simulink model "untitled1"  (R2017b)
settings: Solver=ode4  StartTime=0.0  StopTime=6  FixedStep=Ts  RelTol=1e-3  EnableMultiTasking=on
values from neighbouring files (symbols this model uses):
  init = []    [tunning.m]
  N = 40    [tunning.m]
  Ts = 0.01    [tunning.m]
undefined symbols (not defined in the file or in its folder): data
settings Model: Creator=hqm3yy  LastModifiedBy=tarek
settings OptimizationCC: LifeSpan=inf
settings DebuggingCC: SFUnexpectedBacktrackingDiag=warning  SFNoUnconditionalDefaultTransitionDiag=warning  SFExecutionAtInitializationDiag=none
settings CodeAppCC: StateflowObjectComments=on
settings GRTTargetCC: TargetLangStandard=C89/C90 (ANSI)
settings ConfigComp: CovMetricSettings=dw  CovHtmlReporting=on  CovSaveCumulativeToWorkspaceVar=on  CovSaveSingleToWorkspaceVar=on  CovExternalEMLEnable=off

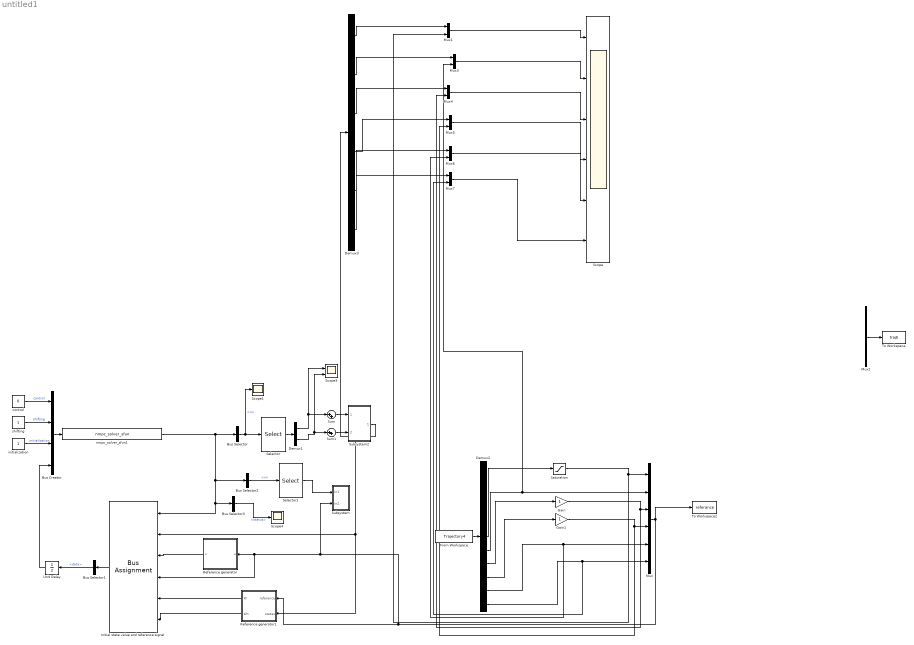
== system untitled1 ==
  Bus Creator : BusCreator  Inputs=4  OutDataTypeStr=Bus: ACADOinput
  Bus Selector : BusSelector  OutputSignals=data.u
  Bus Selector1 : BusSelector  OutputSignals=data
  Bus Selector2 : BusSelector  OutputSignals=data.x
  Bus Selector3 : BusSelector  OutputSignals=status
  Demux1 : Demux  Outputs=2
  Demux2 : Demux  Outputs=11
  Demux3 : Demux  Outputs=6
  From Workspace : FromWorkspace  VariableName=Trajectory4  SampleTime=Ts
  Gain : Gain
  Gain1 : Gain
  Initial state value and reference signal : BusAssignment  AssignedSignals=data.x0,data.y,data.yN,data.W,data.WN
  Mux : Mux  Inputs=6
  Mux{1..7} (7 alike) : Mux  Inputs=2
  Reference generator : Subsystem
      mask help: Simple system simulation.
      mask init:
      | % initialize state values
      mask Display: disp('System');
  Reference generator1 : Subsystem
      mask help: Simple system simulation.
      mask init:
      | % initialize state values
      mask Display: disp('System');
  Saturation : Saturate  UpperLimit=40  LowerLimit=0
  Scope : Scope  NumInputPorts=6
  Scope1 : Scope
  Scope3 : Scope  NumInputPorts=2
  Scope4 : Scope
  Selector : Selector  InputPortWidth=2*N  IndexOptions=Index vector (dialog)  Indices=[1 2]  OutputSizes=2
  Selector1 : Selector  InputPortWidth=(N+1)*6  IndexOptions=Index vector (dialog)  Indices=[1 2 3 4 5 6]  OutputSizes=2
  Subsystem : Subsystem
  Subsystem2 : Subsystem
  Sum : Sum  Inputs=|++
  Sum1 : Sum  Inputs=|++
  To Workspace : ToWorkspace  VariableName=trajE  SampleTime=-1
  To Workspace2 : ToWorkspace  VariableName=referance  SaveFormat=Timeseries  SampleTime=-1
  Unit Delay : UnitDelay  InitialCondition=init  SampleTime=Ts
  control : Constant  Value=0  OutDataTypeStr=int32
  initialization : Constant  OutDataTypeStr=int32
  nmpc_solver_sfun1 : S-Function  FunctionName=nmpc_solver_sfun  SFunctionDeploymentMode=off  EnableBusSupport=off  mask(Legacy Function){SFunctionSpec=nmpc_step(ACADOinput u1[1], ACADOoutput y1[1]), ShowSpec=on}
      mask prompts: ShowSpec "Display function specification"
      mask help:
      | This block allows you to call the legacy functions specified by the following Legacy Code Tool definition:
      | def.SFunctionName = 'nmpc_solver_sfun';
      | def.OutputFcnSpec = 'nmpc_step(ACADOinput u1[1], ACADOoutput y1[1])';
      | def.StartFcnSpec = 'nmpc_initialize( void )';
      | def.TerminateFcnSpec = 'nmpc_cleanup( void )';
      | def.HeaderFiles = {'nmpc_common.h', 'nmpc_solver_sfunction.h'};
      | def.SourceFiles = {'nmpc_solver.c', 'nmpc_integrator.c', 'nmpc_auxiliary_functions.c', 'nmpc_solver_sfunction.c', 'nmpc_qpoases_interface.cpp', 'qpoases\SRC\Bounds.cpp', 'qpoases\SRC\Constraints.cpp', 'qpoases\SRC\CyclingManager.cpp', 'qpoases\SRC\Indexlist.cpp', 'qpoases\SRC\MessageHandling.cpp', 'qpoases\SRC\QProblem.cpp', 'qpoases\SRC\QProblemB.cpp', 'qpoases\SRC\SubjectTo.cpp', 'qpoases\SRC\Utils.cpp', 'qpoases\SRC\EXTRAS\SolutionAnalysis.cpp'};
      | def.IncPaths = {'qpoases', 'qpoases/INCLUDE', 'qpoases/SRC'};
      | def.Options.language = 'C++';
      mask Help: <p>This block was generated automatically by the Legacy Code Tool. For detailed help on this tool, call<a href="matlab:legacy_code('help')"> legacy_code('help')</a>.</p>
      mask Callback ShowSpec:
      | if strcmp(get_param(gcbh, 'ShowSpec'), 'on')
      |   set_param(gcbh, 'MaskDisplay', sprintf('fprintf(''%s'');', get_param(gcbh, 'SFunctionSpec')));
      | else
      |   set_param(gcbh, 'MaskDisplay', sprintf('fprintf(''%s'');', get_param(gcbh, 'FunctionName')));
      | end
      mask Display: fprintf('nmpc_step(ACADOinput u1[1], ACADOoutput y1[1])');
  shifting : Constant  OutDataTypeStr=int32
  wires:
  Initial state value and reference signal/1 -> Bus Selector1/1
  Bus Selector/1 -> Selector/1, Scope1/1  "<u>"
  Selector/1 -> Demux1/1
  Bus Selector1/1 -> Unit Delay/1  "<data>"
  Unit Delay/1 -> Bus Creator/4
  shifting/1 -> Bus Creator/2  "shifting"
  control/1 -> Bus Creator/1  "control"
  initialization/1 -> Bus Creator/3  "initialization"
  Bus Selector2/1 -> Selector1/1  "<x>"
  From Workspace/1 -> Demux2/1
  Bus Creator/1 -> nmpc_solver_sfun1/1
  nmpc_solver_sfun1/1 -> Bus Selector3/1, Initial state value and reference signal/1, Bus Selector2/1, Bus Selector/1
  Reference generator/1(x) -> Initial state value and reference signal/3
  Mux1/1 -> Scope/1
  Demux3/1 -> Mux1/1
  Mux3/1 -> Scope/2
  Demux3/2 -> Mux3/1
  Mux4/1 -> Scope/3
  Demux3/3 -> Mux4/1
  Mux5/1 -> Scope/4
  Demux3/4 -> Mux5/1
  Bus Selector3/1 -> Scope4/1  "<status>"
  Selector1/1 -> Subsystem/1(In1)
  Subsystem2/1(States) -> Initial state value and reference signal/2, Reference generator1/2(" states"), Demux3/1
  Sum/1 -> Subsystem2/1(Steering U1)
  Sum1/1 -> Subsystem2/2(Acceleration U2)
  Reference generator1/2(Wn) -> Initial state value and reference signal/6
  Reference generator1/1(W) -> Initial state value and reference signal/5
  Mux6/1 -> Scope/5
  Demux3/5 -> Mux6/1
  Demux3/6 -> Mux7/1
  Mux7/1 -> Scope/6
  Demux1/1 -> Sum/1, Scope3/1
  Demux1/2 -> Sum1/1, Scope3/2
  Mux/1 -> Subsystem/2(In2), Initial state value and reference signal/4, Reference generator/1(u), Reference generator1/1("referance "), To Workspace2/1
  Gain/1 -> Mux4/2, Mux/3
  Gain1/1 -> Mux5/2, Mux/4
  Mux2/1 -> To Workspace/1
  Saturation/1 -> Mux1/2, Mux/1
  Demux2/6 -> Saturation/1
  Demux2/11 -> Mux7/2, Mux/6
  Demux2/10 -> Mux6/2, Mux/5
  Demux2/9 -> Gain1/1
  Demux2/8 -> Gain/1
  Demux2/7 -> Mux3/2, Mux/2

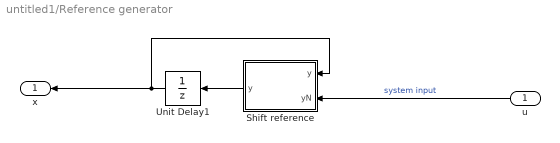
== system untitled1/Reference generator ==
  u : Inport
  Shift reference : MATLAB Function  TreatAsAtomicUnit=on
  Unit Delay1 : UnitDelay  InitialCondition=init.y  SampleTime=Ts
  x : Outport
  wires:
  u/1 -> Shift reference/2(yN)  "system input"
  Shift reference/1(y) -> Unit Delay1/1
  Unit Delay1/1 -> x/1, Shift reference/1("y ")

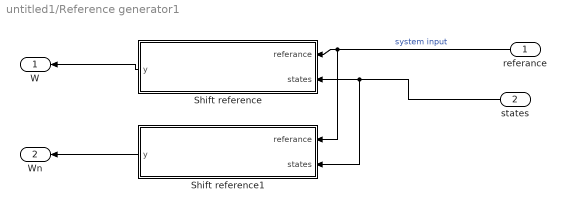
== system untitled1/Reference generator1 ==
  "referance " : Inport
  " states" : Inport  Port=2
  Shift reference : MATLAB Function  TreatAsAtomicUnit=on
  Shift reference1 : MATLAB Function  TreatAsAtomicUnit=on
  W : Outport
  Wn : Outport  Port=2
  wires:
  "referance "/1 -> Shift reference1/1(referance), Shift reference/1(referance)  "system input"
  Shift reference/1(y) -> W/1
  Shift reference1/1(y) -> Wn/1
  " states"/1 -> Shift reference1/2(states), Shift reference/2(states)

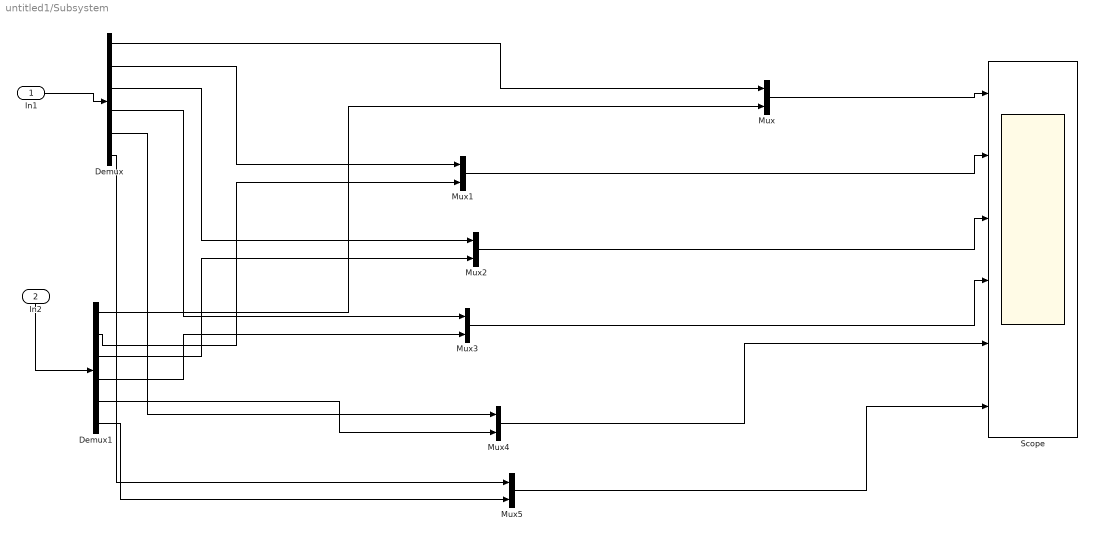
== system untitled1/Subsystem ==
  In1 : Inport
  In2 : Inport  Port=2
  Demux : Demux  Outputs=6
  Demux1 : Demux  Outputs=6
  Mux{,1..5} (6 alike) : Mux  Inputs=2
  Scope : Scope  NumInputPorts=6
  wires:
  In2/1 -> Demux1/1
  In1/1 -> Demux/1
  Mux/1 -> Scope/1
  Mux1/1 -> Scope/2
  Mux3/1 -> Scope/4
  Demux/1 -> Mux/1
  Demux1/1 -> Mux/2
  Demux/2 -> Mux1/1
  Demux1/2 -> Mux1/2
  Demux/3 -> Mux2/1
  Demux1/3 -> Mux2/2
  Demux/4 -> Mux3/1
  Demux1/4 -> Mux3/2
  Mux2/1 -> Scope/3
  Mux4/1 -> Scope/5
  Mux5/1 -> Scope/6
  Demux/5 -> Mux4/1
  Demux1/5 -> Mux4/2
  Demux/6 -> Mux5/1
  Demux1/6 -> Mux5/2

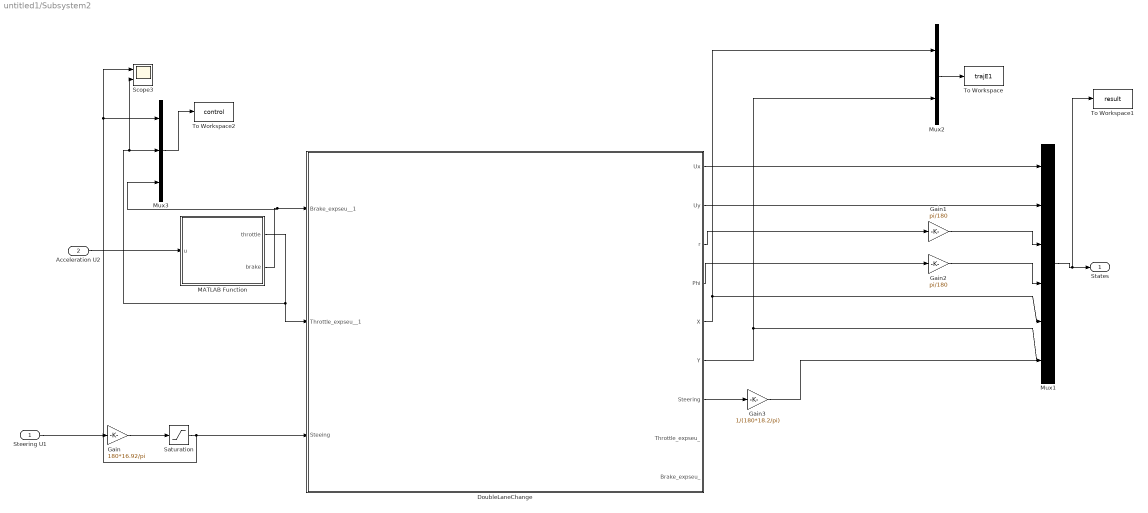
== system untitled1/Subsystem2 ==
  Steering U1 : Inport
  Acceleration U2 : Inport  Port=2
  DoubleLaneChange : Subsystem  Tag=AME2SLCoSim  InitFcn=AMESimLib_initBlock  StartFcn=AMESimLib_startBlock  StopFcn=AMESimLib_stopBlock
      settings: DeleteFcn=AMESimLib_deleteBlock  OpenFcn=AMESimLib_openBlock('AME2SLCoSim')
      mask Display: image(imread('amesim_pix256.png'),[0.4,0.7,0.2,0.2]);disp('Simcenter Amesim co-Sim:\nDoubleLaneChange');port_label('input',1,'Brake_expseu__1');port_label('input',2,'Throttle_expseu__1');port_label('input',3,'Steeing');port_label('output',1,'Ux');port_label('output',2,'Uy');port_label('output',3,'r');port_label('output',4,'Phi');port_label('output',5,'X');port_label('output',6,'Y');port_label('output',7,'Steering');port_label('output',8,'Throttle_expseu_');port_label('output',9,'Brake_expseu_');
  Gain : Gain  Gain=180*16.92/pi
  Gain1 : Gain  Gain=pi/180
  Gain2 : Gain  Gain=pi/180
  Gain3 : Gain  Gain=1/(180*18.2/pi)
  MATLAB Function : MATLAB Function  TreatAsAtomicUnit=on
  Mux1 : Mux  Inputs=6
  Mux2 : Mux  Inputs=2
  Mux3 : Mux  Inputs=3
  Saturation : Saturate  UpperLimit=180  LowerLimit=-180
  Scope3 : Scope  NumInputPorts=2
  To Workspace : ToWorkspace  VariableName=trajE1  SampleTime=-1
  To Workspace1 : ToWorkspace  VariableName=result  SaveFormat=Timeseries  SampleTime=-1
  To Workspace2 : ToWorkspace  VariableName=control  SaveFormat=Timeseries  SampleTime=-1
  States : Outport
  wires:
  Mux1/1 -> To Workspace1/1, States/1
  Mux2/1 -> To Workspace/1
  DoubleLaneChange/1(Ux) -> Mux1/1
  DoubleLaneChange/2(Uy) -> Mux1/2
  DoubleLaneChange/3(r) -> Gain1/1
  DoubleLaneChange/4(Phi) -> Gain2/1
  DoubleLaneChange/5(X) -> Mux2/1, Mux1/5
  DoubleLaneChange/6(Y) -> Mux2/2, Mux1/6
  Saturation/1 -> Scope3/1, Mux3/1, DoubleLaneChange/3(Steeing)
  Acceleration U2/1 -> MATLAB Function/1(u)
  MATLAB Function/1(throttle) -> Scope3/2, Mux3/2, DoubleLaneChange/2(Throttle_expseu__1)
  MATLAB Function/2(brake) -> Mux3/3, DoubleLaneChange/1(Brake_expseu__1)
  Gain/1 -> Saturation/1
  Gain1/1 -> Mux1/3
  Gain2/1 -> Mux1/4
  Steering U1/1 -> Gain/1
  Gain3/1 -> ?
  DoubleLaneChange/7(Steering) -> Gain3/1
  Mux3/1 -> To Workspace2/1

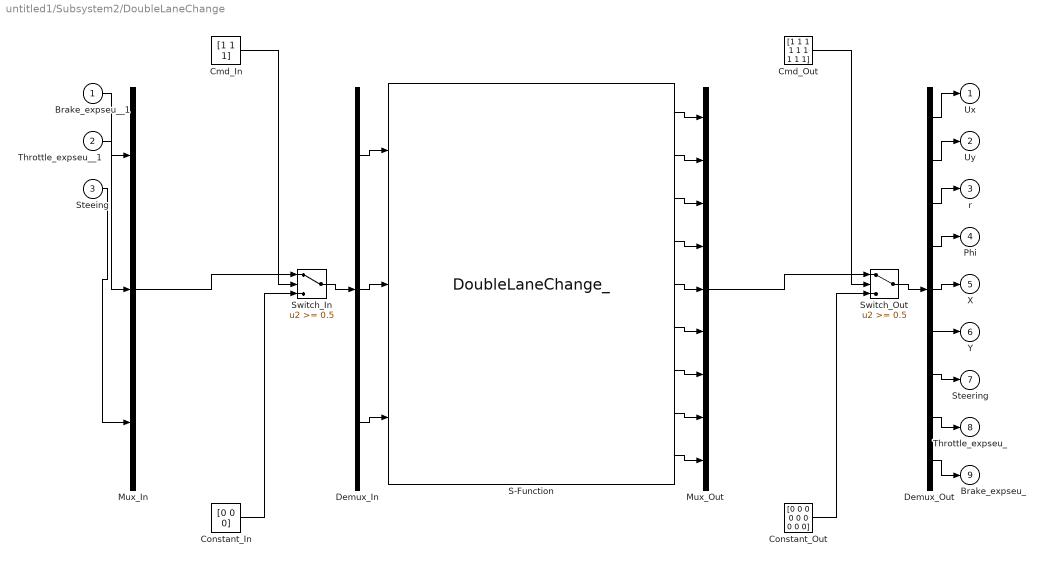
== system untitled1/Subsystem2/DoubleLaneChange ==
  Brake_expseu__1 : Inport
  Throttle_expseu__1 : Inport  Port=2
  Steeing : Inport  Port=3
  Cmd_In : Constant  Value=[1 1 1]
  Cmd_Out : Constant  Value=[1 1 1 1 1 1 1 1 1]
  Constant_In : Constant  Value=[0 0 0]
  Constant_Out : Constant  Value=[0 0 0 0 0 0 0 0 0]
  Demux_In : Demux  Outputs=3
  Demux_Out : Demux  Outputs=9
  Mux_In : Mux  Inputs=3
  Mux_Out : Mux  Inputs=9
  S-Function : S-Function  InitFcn=clear DoubleLaneChange_  StopFcn=clear DoubleLaneChange_  FunctionName=DoubleLaneChange_  Parameters="[0.01;0.001;1e-05;0.05;100;0;0;2;0;2;0.001;0;3] ['Grav           ';'Xg             ';'Zg             ';'Msprung        ';'Msteer         ';'Msp_front      ';'Mwh_front      ';'Msp_rear       ';'Mwh_rear       ';'Isprung_xx     ';'Isprung_yy     ';'Isprung_zz     ';'Isprung_xy     ';'Isprung_xz     ';'Isprung_yz     ';'Zref_front     ';'Zref_rear      ';'wheelbase      ';'track_front    ';'track_rear     ';'Rpinion        ';'Ksusp_front    ';'Ksusp_rear     ';'Rsusp_front    ';'Rsusp_rear     ';'Kantiroll_front';'Kantiroll_rear ';'Rfree          ';'Rroll          ';'Ktire          ';'Rtire          ';'a1             ';'a2             ';'a3             ';'a4             '] [9.8066;1056;375;1300;2;18;18;15;14;250;1000;1300;0;-20;0;75;75;2400;1450;1450;8;21000;21000;2000;1500;30000;20000;0.292;0.291;200000;100;-50;1200;1000;5] [] [] [] []"  SFunctionDeploymentMode=off  EnableBusSupport=off
      mask Display: port_label('output',1,'Ux');port_label('output',2,'Uy');port_label('output',3,'r');port_label('output',4,'Phi');port_label('output',5,'X');port_label('output',6,'Y');port_label('output',7,'Steering');port_label('output',8,'Throttle_expseu_');port_label('output',9,'Brake_expseu_');port_label('input',1,'Brake_expseu__1');port_label('input',2,'Throttle_expseu__1');port_label('input',3,'Steeing');disp('Simcenter Amesim:\n DoubleLaneChange_')
  Switch_In : Switch  Threshold=0.5  SaturateOnIntegerOverflow=on  InputSameDT=on
  Switch_Out : Switch  Threshold=0.5  SaturateOnIntegerOverflow=on  InputSameDT=on
  Ux : Outport
  Uy : Outport  Port=2
  r : Outport  Port=3
  Phi : Outport  Port=4
  X : Outport  Port=5
  Y : Outport  Port=6
  Steering : Outport  Port=7
  Throttle_expseu_ : Outport  Port=8
  Brake_expseu_ : Outport  Port=9
  wires:
  Mux_In/1 -> Switch_In/1
  Cmd_In/1 -> Switch_In/2
  Constant_In/1 -> Switch_In/3
  Switch_In/1 -> Demux_In/1
  Mux_Out/1 -> Switch_Out/1
  Cmd_Out/1 -> Switch_Out/2
  Constant_Out/1 -> Switch_Out/3
  Switch_Out/1 -> Demux_Out/1
  Brake_expseu__1/1 -> Mux_In/1
  Demux_In/1 -> S-Function/1
  Throttle_expseu__1/1 -> Mux_In/2
  Demux_In/2 -> S-Function/2
  Steeing/1 -> Mux_In/3
  Demux_In/3 -> S-Function/3
  Demux_Out/1 -> Ux/1
  S-Function/1 -> Mux_Out/1
  Demux_Out/2 -> Uy/1
  S-Function/2 -> Mux_Out/2
  Demux_Out/3 -> r/1
  S-Function/3 -> Mux_Out/3
  Demux_Out/4 -> Phi/1
  S-Function/4 -> Mux_Out/4
  Demux_Out/5 -> X/1
  S-Function/5 -> Mux_Out/5
  Demux_Out/6 -> Y/1
  S-Function/6 -> Mux_Out/6
  Demux_Out/7 -> Steering/1
  S-Function/7 -> Mux_Out/7
  Demux_Out/8 -> Throttle_expseu_/1
  S-Function/8 -> Mux_Out/8
  Demux_Out/9 -> Brake_expseu_/1
  S-Function/9 -> Mux_Out/9

== matlab function untitled1/Subsystem2/MATLAB Function ==
  data: u input; throttle output; brake output
function [throttle, brake]= fcn(u)
%#codegen

if u > 0
    throttle = abs(u);
    brake = 0;
else
    brake = -0.2*abs(u);
    throttle = 0;
end



end

== matlab function untitled1/Reference generator/Shift reference ==
  data: y input; y output; yN input
function y = shift_reference(y, yN)

NX = 6;
NU = 2;

y = [y(NX+NU+1:end);yN;y(end-NU+1:end)];

== matlab function untitled1/Reference generator1/Shift reference ==
  data: referance input; y output; states input
function y = shift_reference(referance, states)
   
	EUx = abs(referance(1)-states(1)) ;
	EUy = abs(referance(2)-states(2)) ;
	Er  = abs(referance(3)-states(3)) ;
	Ephi= abs(referance(4)-states(4)) ;
	EX  = abs(referance(5)-states(5)) ;
	EY  = abs(referance(6)-states(6)) ;
    
QUx=10*(1+0.1*EUx);
QUy=0;
Qr=10;
Qphi=50;
QX=10*(1+0.1*EX);
QY=20*(1+0.3*EY);

Rs=15;
Rt=20;

w= diag([ QUx  QUy Qr Qphi  QX  QY   Rs  Rt  ]);
 w= reshape (w,1,8*8);
y = w;

== matlab function untitled1/Reference generator1/Shift reference1 ==
  data: referance input; y output; states input
function y = shift_reference(referance, states)
    
	EUx = abs(referance(1)-states(1)) ;
	EUy = abs(referance(2)-states(2)) ;
	Er  = abs(referance(3)-states(3)) ;
	Ephi= abs(referance(4)-states(4)) ;
	EX  = abs(referance(5)-states(5)) ;
	EY  = abs(referance(6)-states(6)) ;

QUx=5;
QUy=0;
Qr=10;
Qphi=50;
QX=30;
QY=20;

Rs=30;
Rt=1;

wn= diag([ QUx  QUy Qr Qphi  QX  QY   ]);
 wn= reshape (wn,1,6*6);
y = wn;
